simulink model "snake_planar_step_11"  (R2020b)
settings: Solver=VariableStepAuto  StartTime=0.0  StopTime=2  RelTol=1e-3
libraries: roblocks x4

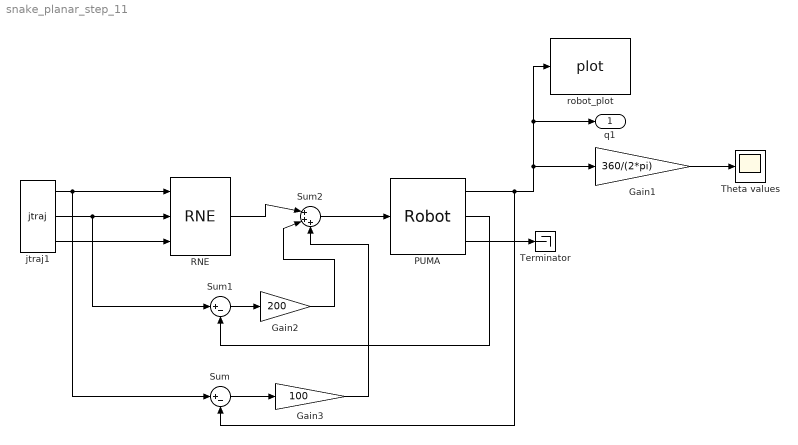
== system snake_planar_step_11 ==
  Gain1 : Gain  Gain=360/(2*pi)
  Gain2 : Gain  Gain=200
  Gain3 : Gain  Gain=100
  PUMA : roblocks/Arm/Robot  robot=snake_planar  q0=[0 0 0 0 0]
  RNE : roblocks/Arm/RNE  robot=snake_planar  grav=[0 0 9.81]
  Sum : Sum  Inputs=|+-
  Sum1 : Sum  Inputs=|+-
  Sum2 : Sum  Inputs=|+++
  Terminator : Terminator
  Theta values : Scope
  jtraj1 : roblocks/Toolbox/jtraj  q0=[0 0 0 0 0]  qf=[pi/2 -pi/4 -pi/4 0 0]  tmax=2  ts=0.02
  robot_plot : roblocks/Arm/plot  robot=snake_planar  fps=5  holdplot=on
  q1 : Outport
  wires:
  PUMA/1 -> Gain1/1, q1/1, robot_plot/1, Sum/2
  Gain1/1 -> Theta values/1
  jtraj1/1 -> RNE/1, Sum/1
  jtraj1/2 -> Sum1/1, RNE/2
  jtraj1/3 -> RNE/3
  Sum1/1 -> Gain2/1
  Sum/1 -> Gain3/1
  Gain3/1 -> Sum2/3
  Gain2/1 -> Sum2/2
  RNE/1 -> Sum2/1
  Sum2/1 -> PUMA/1
  PUMA/2 -> Sum1/2
  PUMA/3 -> Terminator/1
